simulink model "ssupPeuker"  (R2014b)
settings: Solver=ode3  StartTime=0.0  StopTime=.3  FixedStep=.01  RelTol=1e-3
values from neighbouring files (symbols this model uses):
  k = 280    [BslipPeuker.m]
  tMAX = .01*t    [BslipPeuker.m]
  xf = 0    [BslipPeuker.m]
  xinS = xd1.signals.values(end)    [BslipPeuker.m]
  xp = xd.signals.values(end)-(cos(alpha/180*pi)-xpp)    [BslipPeuker.m]
  yinS = yd1.signals.values(end)    [BslipPeuker.m]
  yp = yd.signals.values(end)    [BslipPeuker.m]
undefined symbols (not defined in the file or in its folder): MAX
libraries: simulink x1
settings Model: Creator=hamidreza  LastModifiedBy=hamidreza

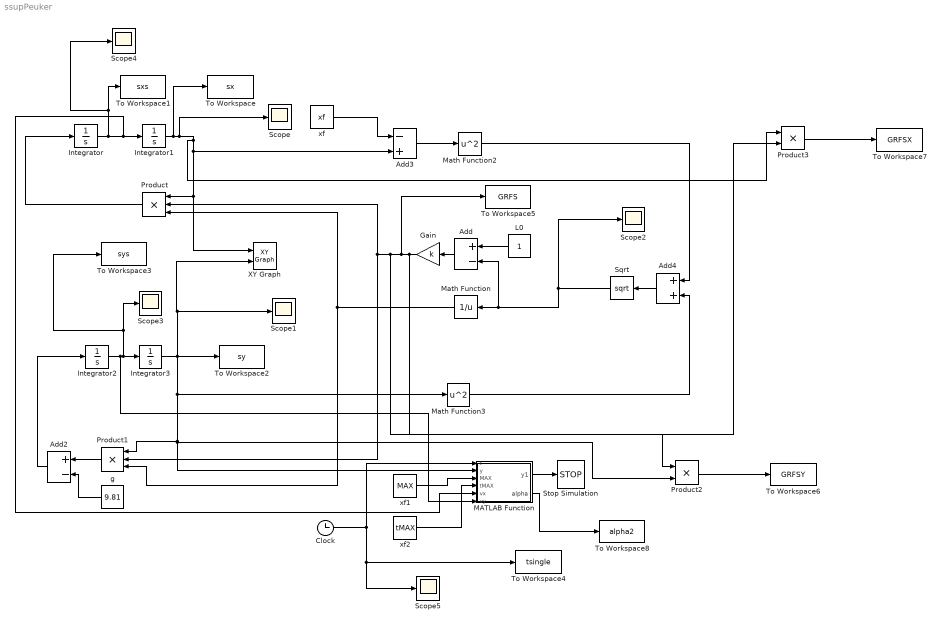
== system ssupPeuker ==
  Add : Sum  Inputs=+-
  Add2 : Sum  Inputs=+-
  Add3 : Sum  Inputs=-+
  Add4 : Sum
  Clock : Clock
  Gain : Gain  Gain=k
  Integrator : Integrator  InitialCondition=xinS
  Integrator1 : Integrator  InitialCondition=xp
  Integrator2 : Integrator  InitialCondition=yinS
  Integrator3 : Integrator  InitialCondition=yp
  L0 : Constant
  MATLAB Function : MATLAB Function  TreatAsAtomicUnit=on
  Math Function : Math  Operator=reciprocal  SaturateOnIntegerOverflow=on
  Math Function2 : Math  Operator=square  SaturateOnIntegerOverflow=on
  Math Function3 : Math  Operator=square  SaturateOnIntegerOverflow=on
  Product : Product  Inputs=3
  Product1 : Product  Inputs=3
  Product2 : Product
  Product3 : Product
  Scope{,1..5} (6 alike) : Scope
      Scope settings: TimeRange=0.17  YMin=-0.102  YMax=-0.088
      Scope1 settings: TimeRange=0.11  YMin=0.965  YMax=0.98
      Scope2 settings: TimeRange=0.14  YMin=0.97  YMax=1.005  SaveName=ScopeData2
      Scope3 settings: SaveName=ScopeData3
      Scope4 settings: TimeRange=1  SaveName=ScopeData4
      Scope5 settings: TimeRange=0.14  YMin=0.97  YMax=1.005  SaveName=ScopeData5
  Sqrt : Sqrt  SaturateOnIntegerOverflow=on
  Stop Simulation : Stop
  To Workspace : ToWorkspace  VariableName=sx  SaveFormat=Structure With Time  SampleTime=-1
  To Workspace1 : ToWorkspace  VariableName=sxs  SaveFormat=Structure With Time  SampleTime=-1
  To Workspace2 : ToWorkspace  VariableName=sy  SaveFormat=Structure With Time  SampleTime=-1
  To Workspace3 : ToWorkspace  VariableName=sys  SaveFormat=Structure With Time  SampleTime=-1
  To Workspace4 : ToWorkspace  VariableName=tsingle  SampleTime=-1
      settings: Save2DSignal=2-D array (concatenate along first dimension)
  To Workspace5 : ToWorkspace  VariableName=GRFS  SaveFormat=Structure With Time  SampleTime=-1
      settings: Save2DSignal=2-D array (concatenate along first dimension)
  To Workspace6 : ToWorkspace  VariableName=GRFSY  SaveFormat=Structure With Time  SampleTime=-1
      settings: Save2DSignal=2-D array (concatenate along first dimension)
  To Workspace7 : ToWorkspace  VariableName=GRFSX  SaveFormat=Structure With Time  SampleTime=-1
      settings: Save2DSignal=2-D array (concatenate along first dimension)
  To Workspace8 : ToWorkspace  VariableName=alpha2  SaveFormat=Structure With Time  SampleTime=-1
      settings: Save2DSignal=2-D array (concatenate along first dimension)
  XY Graph : simulink/Sinks/XY Graph  xmin=-1  xmax=2  ymin=0  ymax=1  st=-1
  g : Constant  Value=9.81
  xf : Constant  Value=xf
  xf1 : Constant  Value=MAX
  xf2 : Constant  Value=tMAX
  wires:
  Integrator/1 -> To Workspace1/1, Scope4/1, MATLAB Function/5(vx), Integrator1/1
  Product/1 -> Integrator/1
  Add/1 -> Gain/1
  Integrator2/1 -> MATLAB Function/6(vy), Scope3/1, To Workspace3/1, Integrator3/1
  Product1/1 -> Add2/1
  g/1 -> Add2/2
  Add2/1 -> Integrator2/1
  xf/1 -> Add3/1
  Add3/1 -> Math Function2/1
  Math Function2/1 -> Add4/1
  Add4/1 -> Sqrt/1
  Sqrt/1 -> Add/2, Math Function/1, Scope2/1
  L0/1 -> Add/1
  Integrator3/1 -> XY Graph/2, Scope1/1, MATLAB Function/2(y), Product2/2, Product1/1, Math Function3/1, To Workspace2/1
  Clock/1 -> To Workspace4/1, Scope5/1, MATLAB Function/1(t)
  MATLAB Function/1(y1) -> Stop Simulation/1
  Math Function3/1 -> Add4/2
  Gain/1 -> Product2/1, To Workspace5/1, Product3/2, Product1/2, Product/2
  Math Function/1 -> Product/3, Product1/3
  Product2/1 -> To Workspace6/1
  Product3/1 -> To Workspace7/1
  Integrator1/1 -> To Workspace/1, Scope/1, Product3/1, Add3/2, Product/1, XY Graph/1
  MATLAB Function/2(alpha) -> To Workspace8/1
  xf1/1 -> MATLAB Function/3(MAX)
  xf2/1 -> MATLAB Function/4(tMAX)

== matlab function ssupPeuker/MATLAB Function ==
  data: t input; y input; MAX input; tMAX input; vx input; vy input; y1 output; alpha output
function [y1,alpha]= fcn(t,y,MAX,tMAX,vx,vy)

    if and(y<=MAX,t>=tMAX)

        gamma=acos(abs(vy)/(sqrt(vx^2+vy^2)));
        alphaa=0.201*gamma;
        alpha=(pi/2-alphaa)/pi*180;
        
        if abs(sin(alpha*pi/180)-y)<.003
            y1=1;
        else
            y1=0;
        end
    
    else
        y1=0;
        alpha=75;
    end
        
end
